simulink model "chap13_4sim"  (Simulink 8.3)
settings: Solver=ode45  SolverMode=SingleTasking  StartTime=0.0  StopTime=20  FixedStep=0.00001  RelTol=1e-3  AbsTol=1e-3
settings Model: Creator=liujk  LastModifiedBy=Administrator  ExtModeTrigMode=oneshot  ExtModeArmWhenConnect=off
settings DataIOCC: LimitDataPoints=off
settings OptimizationCC: BlockReduction=off  BooleanDataType=off
settings DebuggingCC: SaveWithParameterizedLinksMsg=none  SignalResolutionControl=TryResolveAllWithWarning  SolverPrmCheckMsg=none  MultiTaskDSMMsg=warning  MultiTaskCondExecSysMsg=none  FcnCallInpInsideContextMsg=EnableAllAsWarning
settings HardwareCC: TargetUnknown=on
settings RTWCC: IncludeERTFirstTime=on

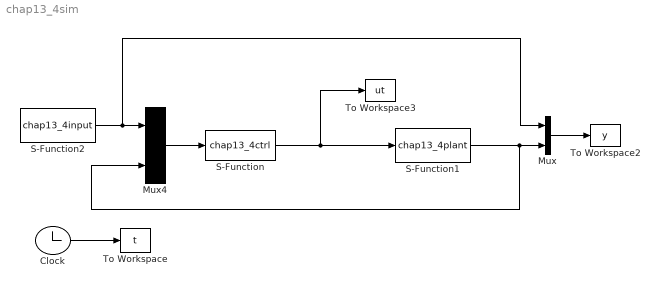
== system chap13_4sim ==
  Clock : Clock
  Mux : Mux  Inputs=2
  Mux4 : Mux  Inputs=2
  S-Function : S-Function  FunctionName=chap13_4ctrl  EnableBusSupport=off
  S-Function1 : S-Function  FunctionName=chap13_4plant  EnableBusSupport=off
  S-Function2 : S-Function  FunctionName=chap13_4input  EnableBusSupport=off
  To Workspace : ToWorkspace  VariableName=t  SampleTime=-1
  To Workspace2 : ToWorkspace  VariableName=y  SampleTime=-1
  To Workspace3 : ToWorkspace  VariableName=ut  SampleTime=-1
  wires:
  Mux4/1 -> S-Function/1
  Mux/1 -> To Workspace2/1
  S-Function1/1 -> Mux/2, Mux4/2
  S-Function2/1 -> Mux4/1, Mux/1
  Clock/1 -> To Workspace/1
  S-Function/1 -> To Workspace3/1, S-Function1/1
